simulink model "v08_full_add"  (R2019b)
settings: Solver=FixedStepAuto  StartTime=0.0  StopTime=inf  FixedStep=1  MaxStep=1  RelTol=1e-3
settings Model: Creator=MARAT  LastModifiedBy=Marat
settings SFSimCC: CustomCodeUndefinedFunction=UseInterfaceOnly

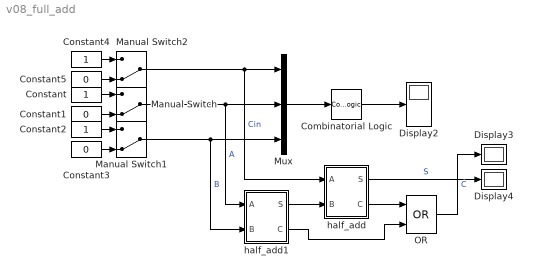
== system v08_full_add ==
  Combinatorial Logic : CombinatorialLogic  TruthTable=[0 0; 0 1; 0 1; 1 0; 0 1; 1 0; 1 0; 1 1]
  Constant : Constant  OutDataTypeStr=boolean
  Constant1 : Constant  Value=0  OutDataTypeStr=boolean
  Constant2 : Constant  OutDataTypeStr=boolean
  Constant3 : Constant  Value=0  OutDataTypeStr=boolean
  Constant4 : Constant  OutDataTypeStr=boolean
  Constant5 : Constant  Value=0  OutDataTypeStr=boolean
  Display2 : Display
  Display3 : Display
  Display4 : Display
  Manual Switch : ManualSwitch  CurrentSetting=0
  Manual Switch1 : ManualSwitch  CurrentSetting=0
  Manual Switch2 : ManualSwitch  CurrentSetting=0
  Mux : Mux  Inputs=3
  OR : Logic  Operator=OR  AllPortsSameDT=off  OutDataTypeStr=boolean
  half_add : Subsystem
  half_add1 : Subsystem
  wires:
  Combinatorial Logic/1 -> Display2/1
  Constant/1 -> Manual Switch/1
  Constant1/1 -> Manual Switch/2
  Constant3/1 -> Manual Switch1/2
  Constant2/1 -> Manual Switch1/1
  Manual Switch/1 -> half_add1/1(A), Mux/2  "A"
  Manual Switch1/1 -> half_add1/2(B), Mux/3  "B"
  Constant4/1 -> Manual Switch2/1
  Constant5/1 -> Manual Switch2/2
  half_add/1(S) -> Display4/1  "S"
  half_add1/1(S) -> half_add/2(B)
  half_add/2(C) -> OR/1
  half_add1/2(C) -> OR/2
  OR/1 -> Display3/1  "C"
  Mux/1 -> Combinatorial Logic/1
  Manual Switch2/1 -> half_add/1(A), Mux/1  "Сin"

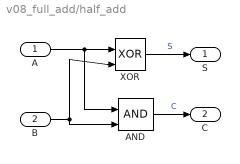
== system v08_full_add/half_add ==
  A : Inport
  B : Inport  Port=2
  AND : Logic  IconShape=distinctive  AllPortsSameDT=off  OutDataTypeStr=boolean
  XOR : Logic  Operator=XOR  IconShape=distinctive  AllPortsSameDT=off  OutDataTypeStr=boolean
  S : Outport
  C : Outport  Port=2
  wires:
  AND/1 -> C/1  "C"
  A/1 -> XOR/1, AND/1
  B/1 -> XOR/2, AND/2
  XOR/1 -> S/1  "S"

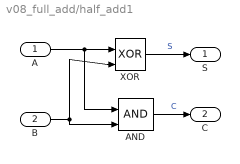
== system v08_full_add/half_add1 ==
  A : Inport
  B : Inport  Port=2
  AND : Logic  IconShape=distinctive  AllPortsSameDT=off  OutDataTypeStr=boolean
  XOR : Logic  Operator=XOR  IconShape=distinctive  AllPortsSameDT=off  OutDataTypeStr=boolean
  S : Outport
  C : Outport  Port=2
  wires:
  XOR/1 -> S/1  "S"
  B/1 -> AND/2, XOR/2
  A/1 -> AND/1, XOR/1
  AND/1 -> C/1  "C"
